simulink model "Powertrain"  (R2025a)
settings: Solver=VariableStepAuto  StartTime=0.0  StopTime=10.0  RelTol=1e-3
values from neighbouring files (symbols this model uses):
  eta_m = 0.4    [variables_procom.m]
  eta_p = O.5    [variables_procom.m]
  eta_r = 0.96    [variables_procom.m]
  Pe = 5    [variables_procom.m]
undefined symbols (not defined in the file or in its folder): nm, Py, Rm, Rme
settings Model: Creator=mathi  LastModifiedBy=mathi

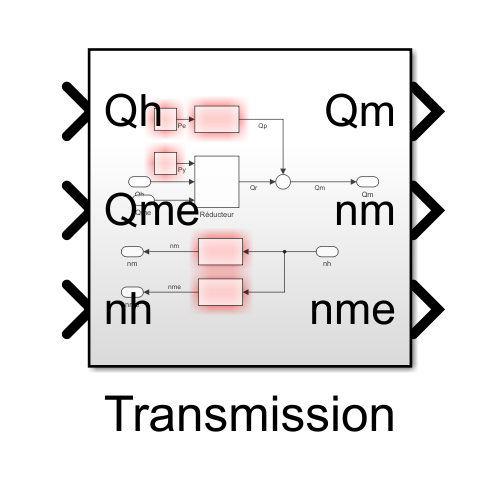
[thumbnail: Simulink's stored preview of the top-level diagram]
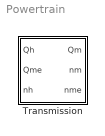
== system Powertrain ==
  Transmission : Subsystem

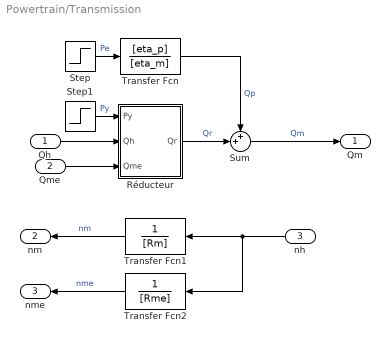
== system Powertrain/Transmission ==
  Qh : Inport
  Qme : Inport  Port=2
  nh : Inport  Port=3
  Réducteur : Subsystem
  Step : Step  Time=0  After=Pe  SampleTime=0
  Step1 : Step  Time=0  After=Py  SampleTime=0
  Sum : Sum  Inputs=++|
  Transfer Fcn : TransferFcn  Numerator=[eta_p]  Denominator=[eta_m]
  Transfer Fcn1 : TransferFcn  Denominator=[Rm]
  Transfer Fcn2 : TransferFcn  Denominator=[Rme]
  Qm : Outport
  nm : Outport  Port=2
  nme : Outport  Port=3
  wires:
  Transfer Fcn/1 -> Sum/1  "Qp"
  Step1/1 -> Réducteur/1(Py)  "Py"
  Qh/1 -> Réducteur/2(Qh)
  nh/1 -> Transfer Fcn2/1, Transfer Fcn1/1
  Transfer Fcn1/1 -> nm/1  "nm"
  Step/1 -> Transfer Fcn/1  "Pe"
  Sum/1 -> Qm/1  "Qm"
  Réducteur/1(Qr) -> Sum/2  "Qr"
  Qme/1 -> Réducteur/3(Qme)
  Transfer Fcn2/1 -> nme/1  "nme"

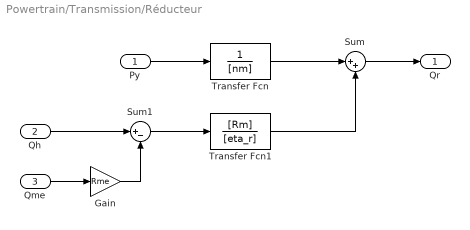
== system Powertrain/Transmission/Réducteur ==
  Py : Inport
  Qh : Inport  Port=2
  Qme : Inport  Port=3
  Gain : Gain  Gain=Rme
  Sum : Sum  Inputs=|++
  Sum1 : Sum  Inputs=|+-
  Transfer Fcn : TransferFcn  Denominator=[nm]
  Transfer Fcn1 : TransferFcn  Numerator=[Rm]  Denominator=[eta_r]
  Qr : Outport
  wires:
  Transfer Fcn/1 -> Sum/1
  Sum/1 -> Qr/1
  Transfer Fcn1/1 -> Sum/2
  Py/1 -> Transfer Fcn/1
  Qme/1 -> Gain/1
  Gain/1 -> Sum1/2
  Qh/1 -> Sum1/1
  Sum1/1 -> Transfer Fcn1/1
